simulink model "TP3"  (R2016a)
settings: Solver=FixedStepAuto  StartTime=0.0  StopTime=4*pi*sqrt(10/9.81)  FixedStep=4*pi*sqrt(10/9.81) / 500  RelTol=1e-6
undefined symbols (not defined in the file): sigbuilder_block
libraries: simulink x2
settings Model: Creator=nsurbayr  LastModifiedBy=nsurbayr

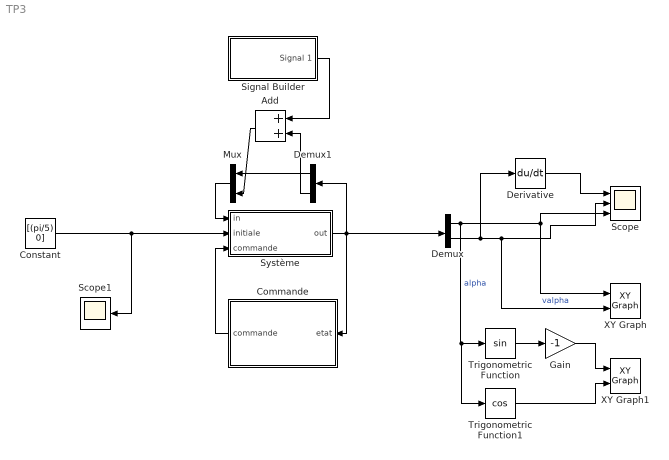
== system TP3 ==
  Add : Sum
  Commande : Subsystem
  Constant : Constant  Value=[(pi/5) 0]  VectorParams1D=off
  Demux : Demux  Outputs=2
  Demux1 : Demux  Outputs=2
  Derivative : Derivative
  Gain : Gain  Gain=-1
  Mux : Mux  Inputs=2
  Scope : Scope  NumInputPorts=3
  Scope1 : Scope
  Signal Builder : Subsystem  Tag=STV Subsys  LoadFcn=sigbuilder_block('load',[437.25 199.5 550.5 399.75 ]);  StartFcn=sigbuilder_block('start');  StopFcn=sigbuilder_block('stop');  ClipboardFcn=sigbuilder_block('clipboard');  mask(Sigbuilder block){}
      mask help: Simulink:masks:SigbuilderBlock_MD
      mask init:
      | if ~strcmp(get_param(bdroot(gcbh),'SimulationStatus'),'stopped') tuvar = sigbuilder_block('maskInit'); end
      settings: CopyFcn=sigbuilder_block('copy');  DeleteFcn=sigbuilder_block('delete');  ModelCloseFcn=sigbuilder_block('modelClose');  PreSaveFcn=sigbuilder_block('preSave');  PauseFcn=sigbuilder_block('pause');  ContinueFcn=sigbuilder_block('continue');  NameChangeFcn=sigbuilder_block('namechange');  OpenFcn=sigbuilder_block('open',[437.25 199.5 550.5 399.75 ]);  CloseFcn=sigbuilder_block('close');
      mask Display: plot(0, 0, 100, 100,[2, 2, 32, 32, 2], [68, 8, 8, 68, 68],[32, 2], [38, 38], [32, 19, 2],[53, 60, 44], [32, 17, 17, 2],[16, 16, 31, 31]);txt = getActiveGroup(gcbh);text(2, 100, txt,'verticalAlignment', 'top');
  Système : Subsystem
  Trigonometric Function : Trigonometry
  Trigonometric Function1 : Trigonometry  Operator=cos
  XY Graph : simulink/Sinks/XY Graph  xmin=-50  xmax=20  ymin=-5  ymax=5  st=-1
  XY Graph1 : simulink/Sinks/XY Graph  xmin=-1  xmax=1  ymin=-1  ymax=1  st=-1
  wires:
  Système/1(out) -> Demux1/1, Commande/1(etat), Demux/1
  Constant/1 -> Scope1/1, Système/2(initiale)
  Demux/2 -> Derivative/1, XY Graph/2, Scope/2  "valpha"
  Demux/1 -> Trigonometric Function1/1, Trigonometric Function/1, XY Graph/1, Scope/3  "alpha"
  Derivative/1 -> Scope/1
  Trigonometric Function/1 -> Gain/1
  Gain/1 -> XY Graph1/1
  Trigonometric Function1/1 -> XY Graph1/2
  Commande/1(commande) -> Système/3(commande)
  Mux/1 -> Système/1(in)
  Demux1/1 -> Mux/1
  Demux1/2 -> Add/2
  Add/1 -> Mux/2
  Signal Builder/1(Signal 1) -> Add/1

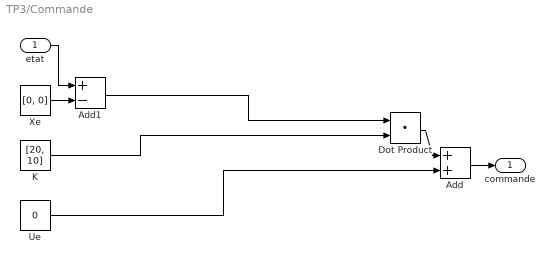
== system TP3/Commande ==
  etat : Inport
  Add : Sum
  Add1 : Sum  Inputs=+-
  Dot Product : DotProduct  InputSameDT=on  OutDataTypeStr=Inherit: Inherit via internal rule
  K : Constant  Value=[20, 10]
  Ue : Constant  Value=0
  Xe : Constant  Value=[0, 0]
  commande : Outport
  wires:
  Add/1 -> commande/1
  Ue/1 -> Add/2
  Dot Product/1 -> Add/1
  K/1 -> Dot Product/2
  Xe/1 -> Add1/2
  etat/1 -> Add1/1
  Add1/1 -> Dot Product/1

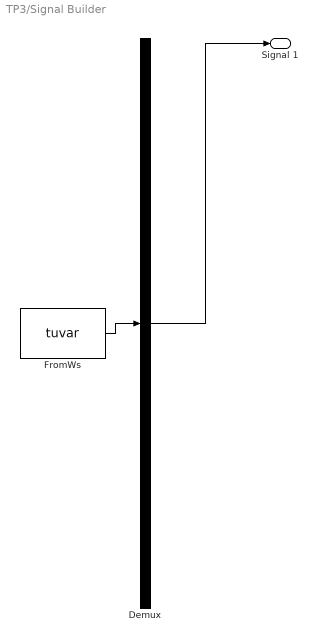
== system TP3/Signal Builder ==
  Demux : Demux  Tag=STV Demux  Outputs=1
  FromWs : FromWorkspace  Tag=STV FromWs  VariableName=tuvar  SampleTime=0
      SigBuilderData=|
      | common.afterFinalStr = 'Extrapolate'
      | common.sampleTime = 0
      | dataSet.timeRange = [0 10]
      | dataSet.name = 'Group 1'
      | sbobj.Groups.Name = 'Group 1'
      | sbobj.Groups.Signals.Name = 'Signal 1'
      | sbobj.Groups.Signals.XData = [0 5.68 5.68 6 6 10]
      | sbobj.Groups.Signals.YData = [0 0 0.79 0.79 0 0]
  Signal 1 : Outport  Tag=STV Outport
  wires:
  Demux/1 -> Signal 1/1
  FromWs/1 -> Demux/1

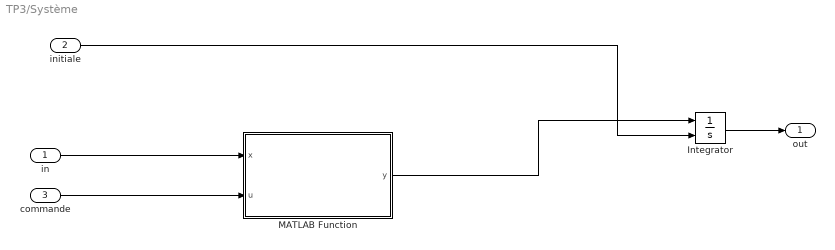
== system TP3/Système ==
  in : Inport
  initiale : Inport  Port=2
  commande : Inport  Port=3
  Integrator : Integrator  InitialConditionSource=external
  MATLAB Function : MATLAB Function  TreatAsAtomicUnit=on
      settings: RTWSystemCode=Inline
  out : Outport
  wires:
  Integrator/1 -> out/1
  initiale/1 -> Integrator/2
  in/1 -> MATLAB Function/1(x)
  commande/1 -> MATLAB Function/2(u)
  MATLAB Function/1(y) -> Integrator/1

== matlab function TP3/Système/MATLAB Function ==
  data: x input; u input; y output
function y = fcn(x,u)

%% Constantes
    g = 9.81;
    l = 10;

%% Calcul
    y = [ x(2) ; ((g*sin(x(1))/l) - (u * cos(x(1))/l)) ];
